simulink model "FFCaracteristic"  (Simulink 7.5)
settings: Solver=ode45  StartTime=0.0  StopTime=1  RelTol=1e-3
libraries: simulink x9, NeuroModelerLibrary x8
settings Model: Creator=Bakhshiev  LastModifiedBy=Bakhshiev

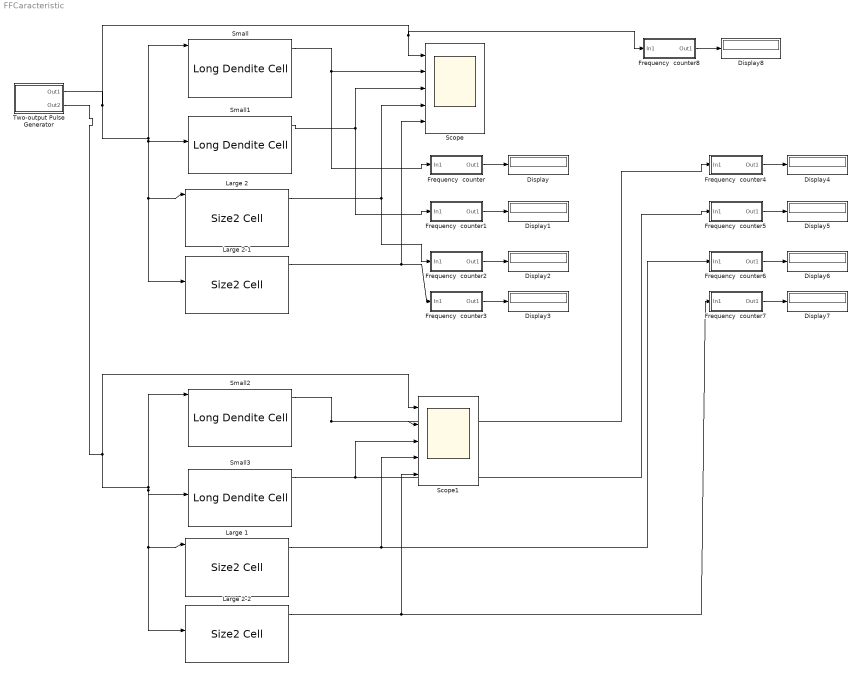
== system FFCaracteristic ==
  Display{,1..8} (9 alike) : Display
  Frequency  counter : Subsystem
  Frequency  counter1 : Subsystem
  Frequency  counter2 : Subsystem
  Frequency  counter3 : Subsystem
  Frequency  counter4 : Subsystem
  Frequency  counter5 : Subsystem
  Frequency  counter6 : Subsystem
  Frequency  counter7 : Subsystem
  Frequency  counter8 : Subsystem
  Large 1 : NeuroModelerLibrary/Sized Cells/Size2 Cell  SystemSampleTime=-1
      link override Synapse: PSMode=1
  Large 2 : NeuroModelerLibrary/Sized Cells/Size2 Cell  SystemSampleTime=-1
  Large 2-1 : NeuroModelerLibrary/Sized Cells/Size2 Cell  SystemSampleTime=-1
  Large 2-2 : NeuroModelerLibrary/Sized Cells/Size2 Cell  SystemSampleTime=-1
      link override Synapse4: PSMode=1
  Scope : Scope  NumInputPorts=5
      settings: YMin=0~-1~-1~0~0  YMax=1~1~1~1~1  MaxDataPoints=50000
  Scope1 : Scope  NumInputPorts=5
      settings: YMin=-0.1~-0.1~-0.1~-0.1~-0.1  YMax=1.1~1.1~1.1~1.1~1.1  MaxDataPoints=50000
  Small : NeuroModelerLibrary/Dendrites Cells/Long Dendite Cell  SystemSampleTime=-1
      link override C2: Value=1
      link override LTZone: T=0.001
      link override Synapse: gamma=1e8  ksi=2
      link override Synapse2: gamma=1e8
      link override Synapse3: gamma=1e8
      link override Synapse4: gamma=1e8
  Small1 : NeuroModelerLibrary/Dendrites Cells/Long Dendite Cell  SystemSampleTime=-1
      link override C2: Value=1
      link override LTZone: T=0.001
      link override Synapse: gamma=1e8
      link override Synapse2: gamma=1e8
      link override Synapse3: gamma=1e8
      link override Synapse4: gamma=1e8  ksi=2
  Small2 : NeuroModelerLibrary/Dendrites Cells/Long Dendite Cell  SystemSampleTime=-1
      link override Synapse: PSMode=1
  Small3 : NeuroModelerLibrary/Dendrites Cells/Long Dendite Cell  SystemSampleTime=-1
      link override Synapse4: PSMode=1
  Two-output Pulse Generator : Subsystem  mask{A=1, P1=20, P2=100, PW=1, ST=0.001, OOn1=0.00, OOff1=1, OOn2=0.0, OOff2=1}
      mask prompts: A "Amplitude"; P1 "Out1: Period (number of samples)"; P2 "Out2: Period (number of samples)"; PW "Pulse Width (number of samples)"; ST "Sample Time"; OOn1 "Out1 On (seconds)"; OOff1 "Out1 Off (seconds)"; OOn2 "Out2 On (seconds)"; OOff2 "Out2 Off (seconds)"
  wires:
  Two-output Pulse Generator/1(Out1) -> Small/1, Large 2/1, Large 2-1/4, Small1/4, Scope/1, Frequency  counter8/1(In1)
  Small/1 -> Frequency  counter/1(In1), Scope/2
  Small1/1 -> Frequency  counter1/1(In1), Scope/3
  Large 2-1/1 -> Scope/5, Frequency  counter3/1(In1)
  Large 2/1 -> Scope/4, Frequency  counter2/1(In1)
  Frequency  counter/1(Out1) -> Display/1
  Frequency  counter1/1(Out1) -> Display1/1
  Frequency  counter2/1(Out1) -> Display2/1
  Frequency  counter3/1(Out1) -> Display3/1
  Two-output Pulse Generator/2(Out2) -> Small2/1, Large 1/1, Large 2-2/4, Small3/4, Scope1/1
  Small2/1 -> Frequency  counter4/1(In1), Scope1/2
  Small3/1 -> Frequency  counter5/1(In1), Scope1/3
  Large 2-2/1 -> Scope1/5, Frequency  counter7/1(In1)
  Large 1/1 -> Scope1/4, Frequency  counter6/1(In1)
  Frequency  counter4/1(Out1) -> Display4/1
  Frequency  counter5/1(Out1) -> Display5/1
  Frequency  counter6/1(Out1) -> Display6/1
  Frequency  counter7/1(Out1) -> Display7/1
  Frequency  counter8/1(Out1) -> Display8/1

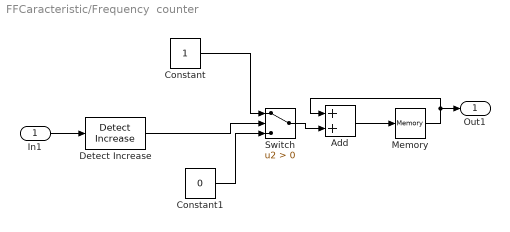
== system FFCaracteristic/Frequency  counter ==
  In1 : Inport
  Add : Sum  OutDataType=fixdt(1, 16)  OutScaling=2^-10
  Constant : Constant  OutDataType=fixdt(1, 16)  OutScaling=2^0
  Constant1 : Constant  Value=0  OutDataType=fixdt(1, 16)  OutScaling=2^0
  Detect Increase : simulink/Logic and Bit Operations/Detect Increase  SystemSampleTime=-1  vinit=0.0
  Memory : Memory
  Switch : Switch  Criteria=u2 > Threshold  OutDataType=fixdt(1, 16)  OutScaling=2^0
  Out1 : Outport
  wires:
  Detect Increase/1 -> Switch/2
  Constant1/1 -> Switch/3
  Constant/1 -> Switch/1
  Switch/1 -> Add/2
  Add/1 -> Memory/1
  Memory/1 -> Add/1, Out1/1
  In1/1 -> Detect Increase/1

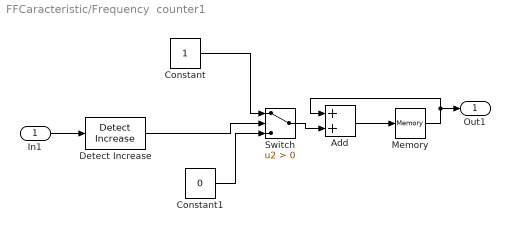
== system FFCaracteristic/Frequency  counter1 ==
  In1 : Inport
  Add : Sum  OutDataType=fixdt(1, 16)  OutScaling=2^-10
  Constant : Constant  OutDataType=fixdt(1, 16)  OutScaling=2^0
  Constant1 : Constant  Value=0  OutDataType=fixdt(1, 16)  OutScaling=2^0
  Detect Increase : simulink/Logic and Bit Operations/Detect Increase  SystemSampleTime=-1  vinit=0.0
  Memory : Memory
  Switch : Switch  Criteria=u2 > Threshold  OutDataType=fixdt(1, 16)  OutScaling=2^0
  Out1 : Outport
  wires:
  Detect Increase/1 -> Switch/2
  Constant1/1 -> Switch/3
  Constant/1 -> Switch/1
  Switch/1 -> Add/2
  Add/1 -> Memory/1
  Memory/1 -> Add/1, Out1/1
  In1/1 -> Detect Increase/1

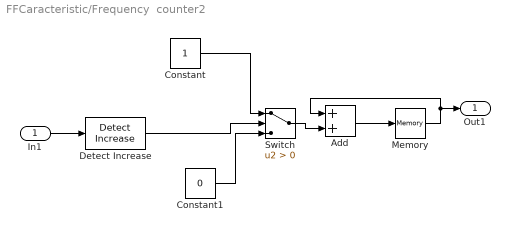
== system FFCaracteristic/Frequency  counter2 ==
  In1 : Inport
  Add : Sum  OutDataType=fixdt(1, 16)  OutScaling=2^-10
  Constant : Constant  OutDataType=fixdt(1, 16)  OutScaling=2^0
  Constant1 : Constant  Value=0  OutDataType=fixdt(1, 16)  OutScaling=2^0
  Detect Increase : simulink/Logic and Bit Operations/Detect Increase  SystemSampleTime=-1  vinit=0.0
  Memory : Memory
  Switch : Switch  Criteria=u2 > Threshold  OutDataType=fixdt(1, 16)  OutScaling=2^0
  Out1 : Outport
  wires:
  Detect Increase/1 -> Switch/2
  Constant1/1 -> Switch/3
  Constant/1 -> Switch/1
  Switch/1 -> Add/2
  Add/1 -> Memory/1
  Memory/1 -> Add/1, Out1/1
  In1/1 -> Detect Increase/1

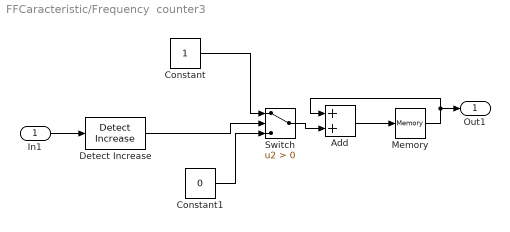
== system FFCaracteristic/Frequency  counter3 ==
  In1 : Inport
  Add : Sum  OutDataType=fixdt(1, 16)  OutScaling=2^-10
  Constant : Constant  OutDataType=fixdt(1, 16)  OutScaling=2^0
  Constant1 : Constant  Value=0  OutDataType=fixdt(1, 16)  OutScaling=2^0
  Detect Increase : simulink/Logic and Bit Operations/Detect Increase  SystemSampleTime=-1  vinit=0.0
  Memory : Memory
  Switch : Switch  Criteria=u2 > Threshold  OutDataType=fixdt(1, 16)  OutScaling=2^0
  Out1 : Outport
  wires:
  Detect Increase/1 -> Switch/2
  Constant1/1 -> Switch/3
  Constant/1 -> Switch/1
  Switch/1 -> Add/2
  Add/1 -> Memory/1
  Memory/1 -> Add/1, Out1/1
  In1/1 -> Detect Increase/1

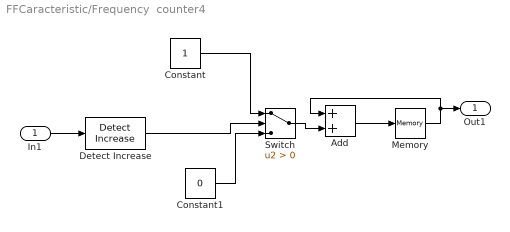
== system FFCaracteristic/Frequency  counter4 ==
  In1 : Inport
  Add : Sum  OutDataType=fixdt(1, 16)  OutScaling=2^-10
  Constant : Constant  OutDataType=fixdt(1, 16)  OutScaling=2^0
  Constant1 : Constant  Value=0  OutDataType=fixdt(1, 16)  OutScaling=2^0
  Detect Increase : simulink/Logic and Bit Operations/Detect Increase  SystemSampleTime=-1  vinit=0.0
  Memory : Memory
  Switch : Switch  Criteria=u2 > Threshold  OutDataType=fixdt(1, 16)  OutScaling=2^0
  Out1 : Outport
  wires:
  Detect Increase/1 -> Switch/2
  Constant1/1 -> Switch/3
  Constant/1 -> Switch/1
  Switch/1 -> Add/2
  Add/1 -> Memory/1
  Memory/1 -> Add/1, Out1/1
  In1/1 -> Detect Increase/1

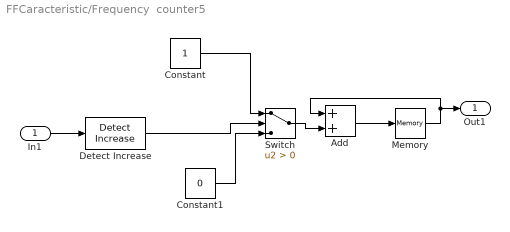
== system FFCaracteristic/Frequency  counter5 ==
  In1 : Inport
  Add : Sum  OutDataType=fixdt(1, 16)  OutScaling=2^-10
  Constant : Constant  OutDataType=fixdt(1, 16)  OutScaling=2^0
  Constant1 : Constant  Value=0  OutDataType=fixdt(1, 16)  OutScaling=2^0
  Detect Increase : simulink/Logic and Bit Operations/Detect Increase  SystemSampleTime=-1  vinit=0.0
  Memory : Memory
  Switch : Switch  Criteria=u2 > Threshold  OutDataType=fixdt(1, 16)  OutScaling=2^0
  Out1 : Outport
  wires:
  Detect Increase/1 -> Switch/2
  Constant1/1 -> Switch/3
  Constant/1 -> Switch/1
  Switch/1 -> Add/2
  Add/1 -> Memory/1
  Memory/1 -> Add/1, Out1/1
  In1/1 -> Detect Increase/1

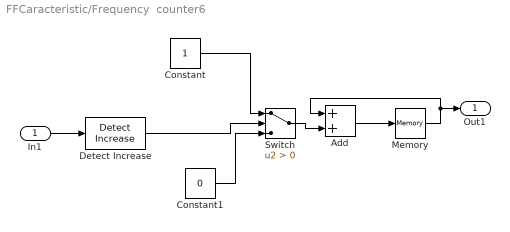
== system FFCaracteristic/Frequency  counter6 ==
  In1 : Inport
  Add : Sum  OutDataType=fixdt(1, 16)  OutScaling=2^-10
  Constant : Constant  OutDataType=fixdt(1, 16)  OutScaling=2^0
  Constant1 : Constant  Value=0  OutDataType=fixdt(1, 16)  OutScaling=2^0
  Detect Increase : simulink/Logic and Bit Operations/Detect Increase  SystemSampleTime=-1  vinit=0.0
  Memory : Memory
  Switch : Switch  Criteria=u2 > Threshold  OutDataType=fixdt(1, 16)  OutScaling=2^0
  Out1 : Outport
  wires:
  Detect Increase/1 -> Switch/2
  Constant1/1 -> Switch/3
  Constant/1 -> Switch/1
  Switch/1 -> Add/2
  Add/1 -> Memory/1
  Memory/1 -> Add/1, Out1/1
  In1/1 -> Detect Increase/1

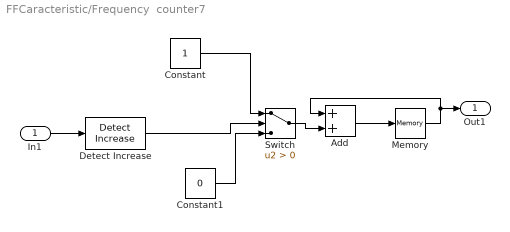
== system FFCaracteristic/Frequency  counter7 ==
  In1 : Inport
  Add : Sum  OutDataType=fixdt(1, 16)  OutScaling=2^-10
  Constant : Constant  OutDataType=fixdt(1, 16)  OutScaling=2^0
  Constant1 : Constant  Value=0  OutDataType=fixdt(1, 16)  OutScaling=2^0
  Detect Increase : simulink/Logic and Bit Operations/Detect Increase  SystemSampleTime=-1  vinit=0.0
  Memory : Memory
  Switch : Switch  Criteria=u2 > Threshold  OutDataType=fixdt(1, 16)  OutScaling=2^0
  Out1 : Outport
  wires:
  Detect Increase/1 -> Switch/2
  Constant1/1 -> Switch/3
  Constant/1 -> Switch/1
  Switch/1 -> Add/2
  Add/1 -> Memory/1
  Memory/1 -> Add/1, Out1/1
  In1/1 -> Detect Increase/1

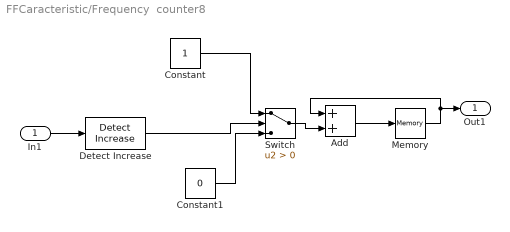
== system FFCaracteristic/Frequency  counter8 ==
  In1 : Inport
  Add : Sum  OutDataType=fixdt(1, 16)  OutScaling=2^-10
  Constant : Constant  OutDataType=fixdt(1, 16)  OutScaling=2^0
  Constant1 : Constant  Value=0  OutDataType=fixdt(1, 16)  OutScaling=2^0
  Detect Increase : simulink/Logic and Bit Operations/Detect Increase  SystemSampleTime=-1  vinit=0.0
  Memory : Memory
  Switch : Switch  Criteria=u2 > Threshold  OutDataType=fixdt(1, 16)  OutScaling=2^0
  Out1 : Outport
  wires:
  Detect Increase/1 -> Switch/2
  Constant1/1 -> Switch/3
  Constant/1 -> Switch/1
  Switch/1 -> Add/2
  Add/1 -> Memory/1
  Memory/1 -> Add/1, Out1/1
  In1/1 -> Detect Increase/1

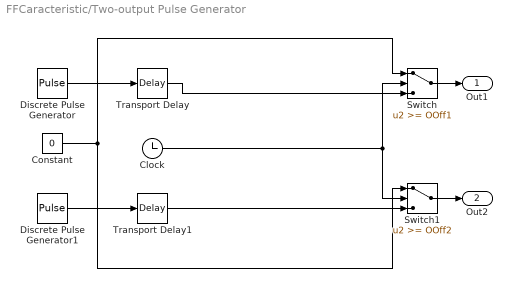
== system FFCaracteristic/Two-output Pulse Generator ==
  Clock : Clock
      settings: Decimation=10
  Constant : Constant  Value=0
  Discrete Pulse Generator : DiscretePulseGenerator  Amplitude=A  Period=P1  PulseWidth=PW  PhaseDelay=0  SampleTime=ST
  Discrete Pulse Generator1 : DiscretePulseGenerator  Amplitude=A  Period=P2  PulseWidth=PW  PhaseDelay=0  SampleTime=ST
  Switch : Switch  Threshold=OOff1  SaturateOnIntegerOverflow=on  InputSameDT=on
  Switch1 : Switch  Threshold=OOff2  SaturateOnIntegerOverflow=on  InputSameDT=on
  Transport Delay : TransportDelay  DelayTime=OOn1
  Transport Delay1 : TransportDelay  DelayTime=OOn2
  Out1 : Outport  InitialOutput=0
  Out2 : Outport  Port=2  InitialOutput=0
  wires:
  Discrete Pulse Generator/1 -> Transport Delay/1
  Constant/1 -> Switch/1, Switch1/1
  Discrete Pulse Generator1/1 -> Transport Delay1/1
  Transport Delay1/1 -> Switch1/3
  Transport Delay/1 -> Switch/3
  Clock/1 -> Switch/2, Switch1/2
  Switch/1 -> Out1/1
  Switch1/1 -> Out2/1
